simulink model "Controller_Design_for_Position_Control_simulink"  (R2020b)
settings: Solver=VariableStepAuto  StartTime=0.0  StopTime=150.0  RelTol=1e-3
values from neighbouring files (symbols this model uses):
  C1 = 10    [Controller_Design_for_Position_Control.m]    (also in PI_Controller_Design_for_Speed_Control.m)
  C2 = 0.6    [Controller_Design_for_Position_Control.m]    (also in PI_Controller_Design_for_Speed_Control.m)
  Ki = 100    [Controller_Design_for_Position_Control.m]    (also in PI_Controller_Design_for_Speed_Control.m = 3.04)
  Kp = 200    [Controller_Design_for_Position_Control.m]    (also in PI_Controller_Design_for_Speed_Control.m = 0.215)
settings Model: Creator=marco  LastModifiedBy=marco

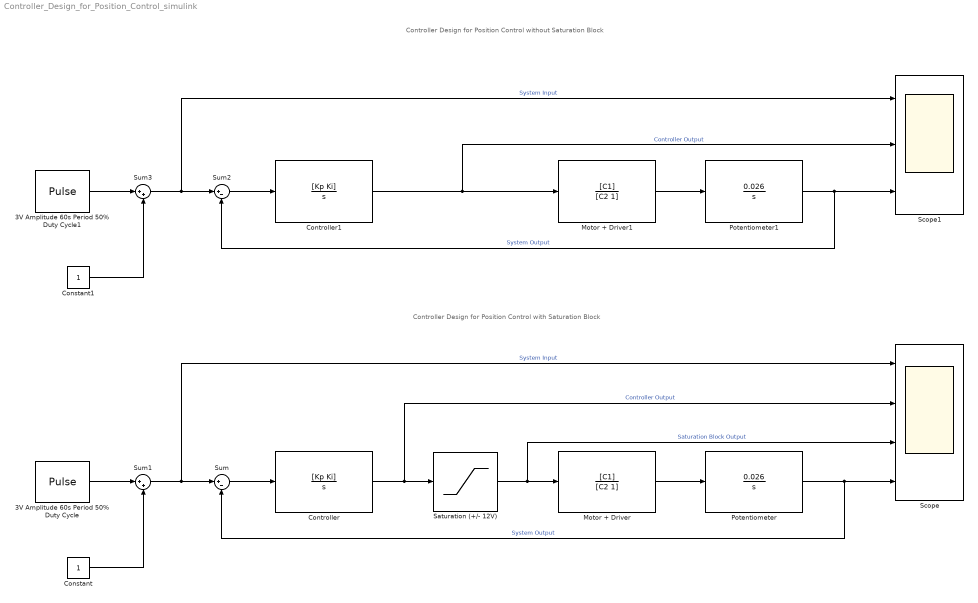
== system Controller_Design_for_Position_Control_simulink ==
  note: Controller Design for Position Control without Saturation Block
  note: Controller Design for Position Control with Saturation Block
  3V Amplitude 60s Period 50% Duty Cycle : DiscretePulseGenerator  PulseType=Time based  Amplitude=3  Period=60  PulseWidth=50
  3V Amplitude 60s Period 50% Duty Cycle1 : DiscretePulseGenerator  PulseType=Time based  Amplitude=3  Period=60  PulseWidth=50
  Constant : Constant
  Constant1 : Constant
  Controller : TransferFcn  Numerator=[Kp Ki]  Denominator=[1 0]
  Controller1 : TransferFcn  Numerator=[Kp Ki]  Denominator=[1 0]
  Motor + Driver : TransferFcn  Numerator=[C1]  Denominator=[C2 1]
  Motor + Driver1 : TransferFcn  Numerator=[C1]  Denominator=[C2 1]
  Potentiometer : TransferFcn  Numerator=[0.026]  Denominator=[1 0]
  Potentiometer1 : TransferFcn  Numerator=[0.026]  Denominator=[1 0]
  Saturation (+/- 12V) : Saturate  UpperLimit=12  LowerLimit=-12
  Scope : Scope  NumInputPorts=4
  Scope1 : Scope  NumInputPorts=3
  Sum : Sum  Inputs=|+-
  Sum1 : Sum  Inputs=|++
  Sum2 : Sum  Inputs=|+-
  Sum3 : Sum  Inputs=|++
  wires:
  Sum/1 -> Controller/1
  Constant/1 -> Sum1/2
  Potentiometer/1 -> Sum/2, Scope/4  "System Output"
  Sum1/1 -> Sum/1, Scope/1  "System Input"
  Controller/1 -> Scope/2, Saturation (+/- 12V)/1  "Controller Output"
  Motor + Driver/1 -> Potentiometer/1
  3V Amplitude 60s Period 50% Duty Cycle/1 -> Sum1/1
  Saturation (+/- 12V)/1 -> Scope/3, Motor + Driver/1  "Saturation Block Output"
  Motor + Driver1/1 -> Potentiometer1/1
  Constant1/1 -> Sum3/2
  Sum3/1 -> Scope1/1, Sum2/1  "System Input"
  Sum2/1 -> Controller1/1
  Potentiometer1/1 -> Sum2/2, Scope1/3  "System Output"
  3V Amplitude 60s Period 50% Duty Cycle1/1 -> Sum3/1
  Controller1/1 -> Scope1/2, Motor + Driver1/1  "Controller Output"
